simulink model "ec"  (R2021b)
settings: Solver=VariableStepAuto  StartTime=0.0  StopTime=10  RelTol=1e-3
settings Model: Creator=Alumno103  LastModifiedBy=Alumno103

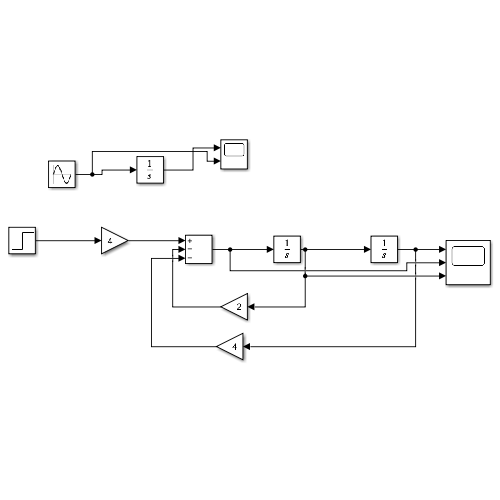
[thumbnail: Simulink's stored preview of the top-level diagram]
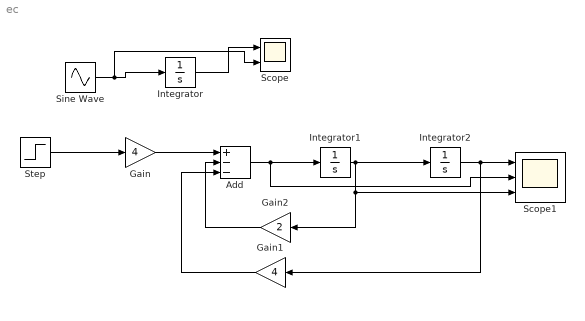
== system ec ==
  Add : Sum  Inputs=+--
  Gain : Gain  Gain=4
  Gain1 : Gain  Gain=4
  Gain2 : Gain  Gain=2
  Integrator : Integrator  InitialCondition=5
  Integrator1 : Integrator
  Integrator2 : Integrator
  Scope : Scope  NumInputPorts=2
  Scope1 : Scope  NumInputPorts=3
  Sine Wave : Sin  Frequency=5  SampleTime=0
  Step : Step  SampleTime=0
  wires:
  Sine Wave/1 -> Scope/2, Integrator/1
  Integrator/1 -> Scope/1
  Step/1 -> Gain/1
  Gain/1 -> Add/1
  Add/1 -> Scope1/2, Integrator1/1
  Integrator1/1 -> Gain2/1, Scope1/3, Integrator2/1
  Integrator2/1 -> Gain1/1, Scope1/1
  Gain2/1 -> Add/2
  Gain1/1 -> Add/3
